simulink model "pci1756"  (R2016b)
settings: Solver=ode4  StartTime=0.0  StopTime=inf  FixedStep=0.002  RelTol=1e-3  EnableMultiTasking=on
settings Model: SimulationMode=external  Creator=Administrator  LastModifiedBy=Administrator
settings SolverCC: EnableConcurrentExecution=on
settings DataIOCC: SaveFormat=StructureWithTime
settings OptimizationCC: BlockReduction=off  OptimizeBlockIOStorage=off  BufferReuse=off  GlobalBufferReuse=off  ExpressionFolding=off  LocalBlockOutputs=off
settings HardwareCC: ProdBitPerPointer=32  ProdBitPerSizeT=32  ProdBitPerPtrDiffT=32  ProdLargestAtomicFloat=None  ProdWordSize=32  ProdLongLongMode=on  ProdHWDeviceType=Generic->32-bit x86 compatible
settings RTWCC: SystemTargetFile=slrt.tlc  TemplateMakefile=slrt_default_tmf  Description=Simulink Real-Time  RTWCompilerOptimization=on

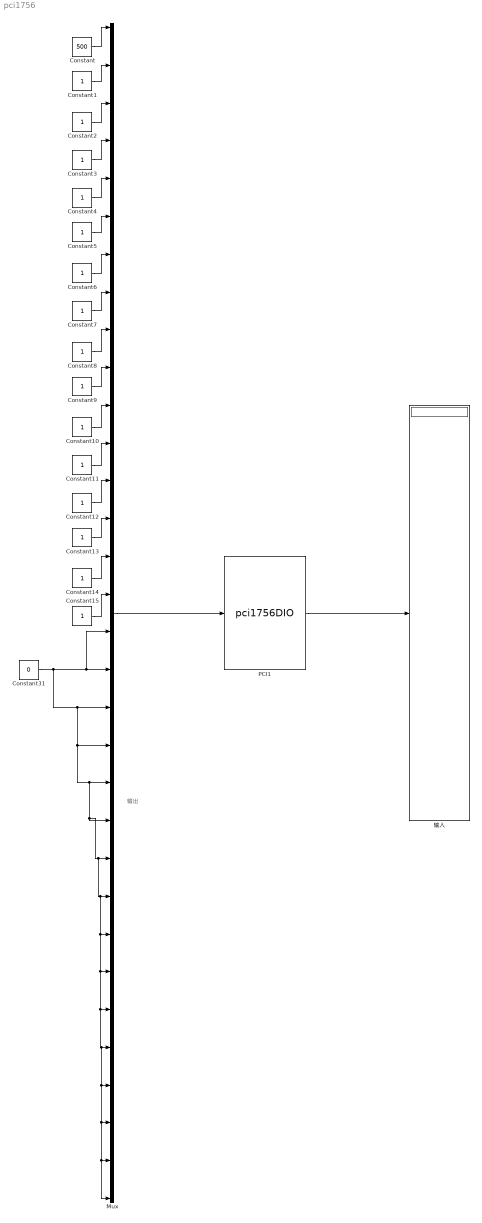
== system pci1756 ==
  note: 输出
  Constant : Constant  Value=500
  Constant{1..15} (15 alike) : Constant
  Constant31 : Constant  Value=0
  Mux : Mux  Inputs=32
  PCI1 : S-Function  FunctionName=pci1756DIO  Parameters=[SampleTime SampleOffset], SLOT  SFunctionDeploymentMode=off  EnableBusSupport=off  mask(PCI1756){Sample=0.002, SLOT=-1}
      mask prompts: Sample "Sample time:"
      mask help:
      | PCI-1756
      | Advantech
      | Digital Input&Output
      mask init:
      | SampleTime =0.002; SampleOffset=0;
      mask Display:
      | disp('PCI1756\nDigital output&input\n');
      | port_label('input',1,'32');
      | 
      | port_label('output',1,'32');
  输入 : Display
  wires:
  Constant/1 -> Mux/1
  Constant1/1 -> Mux/2
  Constant2/1 -> Mux/3
  Constant3/1 -> Mux/4
  Constant4/1 -> Mux/5
  Constant5/1 -> Mux/6
  Constant6/1 -> Mux/7
  Constant7/1 -> Mux/8
  Constant8/1 -> Mux/9
  Constant9/1 -> Mux/10
  Constant10/1 -> Mux/11
  Constant11/1 -> Mux/12
  Constant12/1 -> Mux/13
  Constant13/1 -> Mux/14
  Constant14/1 -> Mux/15
  Constant15/1 -> Mux/16
  Mux/1 -> PCI1/1
  PCI1/1 -> 输入/1
  Constant31/1 -> Mux/32, Mux/31, Mux/30, Mux/29, Mux/28, Mux/27, Mux/26, Mux/25, Mux/24, Mux/23, Mux/22, Mux/21, Mux/20, Mux/19, Mux/17, Mux/18
